simulink model "E_2"  (R2020a)
settings: Solver=VariableStepAuto  StartTime=0.0  StopTime=10.0  RelTol=1e-3
settings Model: Creator=Santiago  LastModifiedBy=Santiago

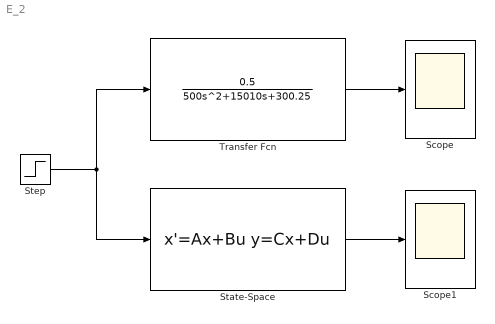
== system E_2 ==
  Scope : Scope
  Scope1 : Scope
  State-Space : StateSpace  A=[-0.02 0.005;-0.1 -30]  B=[0;0.2]  C=[1 0]  D=0  InitialCondition=0
  Step : Step  SampleTime=0
  Transfer Fcn : TransferFcn  Numerator=[0.5]  Denominator=[500 15010 300.25]
  wires:
  Step/1 -> State-Space/1, Transfer Fcn/1
  Transfer Fcn/1 -> Scope/1
  State-Space/1 -> Scope1/1
